simulink model "A_Justo_SCHFV_slx_Track"  (R2019a)
settings: Solver=VariableStepAuto  StartTime=0.0  StopTime=tfinal  MaxStep=maxstepsize  RelTol=1e-3  EnableMultiTasking=on
values from neighbouring files (symbols this model uses):
  acc1 = 0    [A_Justo_SCHFV_m_IV.m]    (also in A_Justo_SCHFV_m_Track.m)
  acc2 = 0    [A_Justo_SCHFV_m_IV.m]    (also in A_Justo_SCHFV_m_Track.m)
  add_u_1 = zeros(N,1); add_u_1(acc1) = 1    [A_Justo_SCHFV_m_Track.m]
  add_u_2 = zeros(N,1)    [A_Justo_SCHFV_m_Track.m]
  aini = 0    [A_Justo_SCHFV_m_UFHDV_Design.m]
  B = [0; 0; 0; 0; 1/Tau_A]    [A_Justo_SCHFV_m_Control_Sensitivity.m]    (also in A_Justo_SCHFV_m_UFHDV_Design.m; TransferFunctionPROP.m)
  IDM_Amax = IDM_Amax(acc1+n1,acc1+n1)    [TransferFunctionPROP.m]
  IDM_Bmax = IDM_Bmax(acc1+n1,acc1+n1)    [TransferFunctionPROP.m]
  IDM_Delta = IDM_Delta(acc1+n1)    [TransferFunctionPROP.m]
  IDM_H0 = IDM_H0(acc1+n1)    [TransferFunctionPROP.m]
  IDM_T = normrnd(IDM_t,IDM_ts)    [A_Justo_SCHFV_m_Control_Sensitivity.m]    (also in A_Justo_SCHFV_m_Track.m = IDM_Tind; A_Justo_SCHFV_m_UFHDV_Design.m; TransferFunctionPROP.m = IDM_T(acc1+n1,acc1+n1))
  IDM_V0 = IDM_V0(acc1+n1)    [TransferFunctionPROP.m]
  kgain = 0.02    [A_Justo_SCHFV_m_Track.m]    (also in A_Justo_SCHFV_m_UFHDV_Design.m)
  Lini = Lind    [A_Justo_SCHFV_m_Track.m]    (also in A_Justo_SCHFV_m_UFHDV_Design.m = sum(normrnd(l,ls,1,n)))
  N = 11    [A_Justo_SCHFV_m_IV.m]    (also in A_Justo_SCHFV_m_Track.m)
  n1 = 0    [A_Justo_SCHFV_m_IV.m]    (also in A_Justo_SCHFV_m_Track.m = 10)
  R = d/(2*pi)    (= 31.8309886184)    [A_Justo_SCHFV_m_IV.m]    (also in A_Justo_SCHFV_m_Track.m)
  Sacc = diag(isACC)    [A_Justo_SCHFV_m_Track.m]
  sep_a_A_1 = zeros(1,N); sep_a_A_1(acc1) = 1    [A_Justo_SCHFV_m_Track.m]
  sep_a_A_2 = zeros(1,N)    [A_Justo_SCHFV_m_Track.m]
  sep_a_H_1 = zeros(1,N); sep_a_H_1(acc1+n1) = 1    [A_Justo_SCHFV_m_Track.m]
  sep_a_H_2 = zeros(1,N)    [A_Justo_SCHFV_m_Track.m]
  sep_h_H_1 = zeros(1,N); sep_h_H_1(acc1+1) = 1    [A_Justo_SCHFV_m_Track.m]
  sep_h_H_2 = zeros(1,N)    [A_Justo_SCHFV_m_Track.m]
  sep_v_A_1 = zeros(1,N); sep_v_A_1(acc1) = 1    [A_Justo_SCHFV_m_Track.m]
  sep_v_A_2 = zeros(1,N)    [A_Justo_SCHFV_m_Track.m]
  sep_v_H_1 = zeros(1,N); sep_v_H_1(acc1+n1) = 1    [A_Justo_SCHFV_m_Track.m]
  sep_v_H_2 = zeros(1,N)    [A_Justo_SCHFV_m_Track.m]
  Sidm = diag(isIDM)    [A_Justo_SCHFV_m_IV.m]    (also in A_Justo_SCHFV_m_Track.m)
  Smit = diag(isMIT)    [A_Justo_SCHFV_m_IV.m]    (also in A_Justo_SCHFV_m_Track.m)
  T_s_0 = 60    [A_Justo_SCHFV_m_Track.m]
  v_r_0 = 30/3.6    (= 8.33333333333)    [A_Justo_SCHFV_m_Control_Sensitivity.m]    (also in A_Justo_SCHFV_m_Track.m = 5.55555555556; A_Justo_SCHFV_m_UFHDV_Design.m = 2.77777777778)
  vini = 0    [A_Justo_SCHFV_m_UFHDV_Design.m]
undefined symbols (not defined in the file or in its folder): Bv, IDM_iSqab, iTau, MITSIM_a_Free_bra_high, MITSIM_a_Free_bra_low, MITSIM_a_Free_bra_mid, MITSIM_a_Free_bra_midhigh, MITSIM_a_Free_bra_midlow, MITSIM_a_Free_thr_high, MITSIM_a_Free_thr_low, MITSIM_a_Free_thr_mid, MITSIM_Alpha_bra, MITSIM_Alpha_thr, MITSIM_Beta_bra, MITSIM_Beta_thr, MITSIM_Gamma_bra, MITSIM_Gamma_thr, MITSIM_T_lower, MITSIM_T_upper, Tau, thini
settings Model: Creator=arnaudoria  LastModifiedBy=Sander
settings DataIOCC: LimitDataPoints=on  ReturnWorkspaceOutputs=off
settings OptimizationCC: LifeSpan=inf
settings DebuggingCC: AllowSymbolicDim=off  SFUnexpectedBacktrackingDiag=warning  SFNoUnconditionalDefaultTransitionDiag=warning  SFExecutionAtInitializationDiag=none  ArithmeticOperatorsInVariantConditions=warning
settings ModelReferenceCC: PropagateSignalLabelsOutOfModel=off
settings SFSimCC: SimUseLocalCustomCode=off
settings RTWCC: RTWUseLocalCustomCode=off
settings CodeAppCC: StateflowObjectComments=on
settings GRTTargetCC: TargetLangStandard=C89/C90 (ANSI)
settings ConfigComp: CovMetricSettings=dw  CovHtmlReporting=on  CovSaveCumulativeToWorkspaceVar=on  CovSaveSingleToWorkspaceVar=on  CovExternalEMLEnable=off

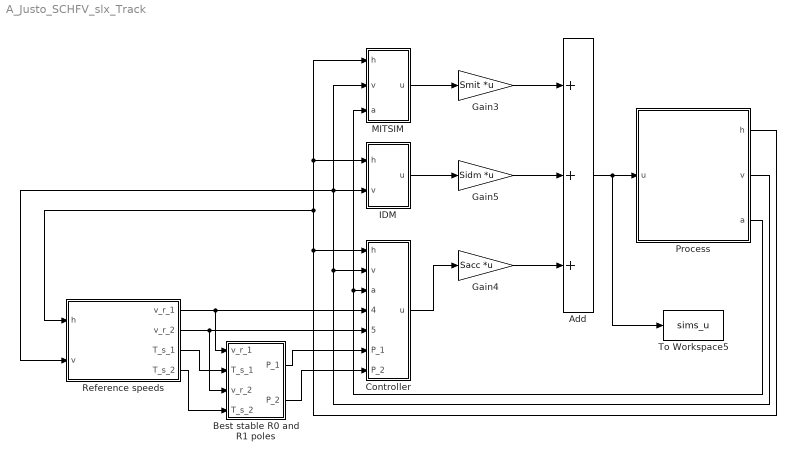
== system A_Justo_SCHFV_slx_Track ==
  Add : Sum  Inputs=+++
  Best stable R0 and R1 poles : Subsystem
  Controller : Subsystem
  Gain3 : Gain  Gain=Smit  Multiplication=Matrix(K*u)
  Gain4 : Gain  Gain=Sacc  Multiplication=Matrix(K*u)
  Gain5 : Gain  Gain=Sidm  Multiplication=Matrix(K*u)
  IDM : Subsystem
  MITSIM : Subsystem
  Process : Subsystem
  Reference speeds : Subsystem
  To Workspace5 : ToWorkspace  VariableName=sims_u  SampleTime=-1
  wires:
  Process/1(h) -> Reference speeds/1(h), IDM/1(h), MITSIM/1(h), Controller/1(h)
  Process/2(v) -> Reference speeds/2(v), MITSIM/2(v), IDM/2(v), Controller/2(v)
  Process/3(a) -> MITSIM/3(a), Controller/3(a)
  Controller/1(u) -> Gain4/1
  Gain4/1 -> Add/3
  Add/1 -> Process/1(u), To Workspace5/1
  Gain5/1 -> Add/2
  IDM/1(u) -> Gain5/1
  MITSIM/1(u) -> Gain3/1
  Gain3/1 -> Add/1
  Reference speeds/1(v_r_1) -> Controller/4(v_r_1), Best stable R0 and R1 poles/1(v_r_1)
  Best stable R0 and R1 poles/1(P_1) -> Controller/6(P_1)
  Reference speeds/2(v_r_2) -> Best stable R0 and R1 poles/3(v_r_2), Controller/5(v_r_2)
  Best stable R0 and R1 poles/2(P_2) -> Controller/7(P_2)
  Reference speeds/3(T_s_1) -> Best stable R0 and R1 poles/2(T_s_1)
  Reference speeds/4(T_s_2) -> Best stable R0 and R1 poles/4(T_s_2)

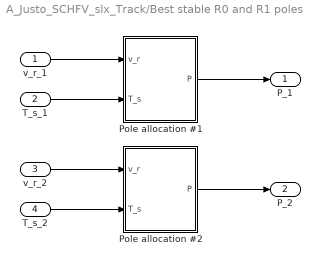
== system A_Justo_SCHFV_slx_Track/Best stable R0 and R1 poles ==
  v_r_1 : Inport
  T_s_1 : Inport  Port=2
  v_r_2 : Inport  Port=3
  T_s_2 : Inport  Port=4
  Pole allocation #1 : MATLAB Function  TreatAsAtomicUnit=on
  Pole allocation #2 : MATLAB Function  TreatAsAtomicUnit=on
  P_1 : Outport
  P_2 : Outport  Port=2
  wires:
  v_r_1/1 -> Pole allocation #1/1(v_r)
  Pole allocation #1/1(P) -> P_1/1
  T_s_1/1 -> Pole allocation #1/2(T_s)
  Pole allocation #2/1(P) -> P_2/1
  T_s_2/1 -> Pole allocation #2/2(T_s)
  v_r_2/1 -> Pole allocation #2/1(v_r)

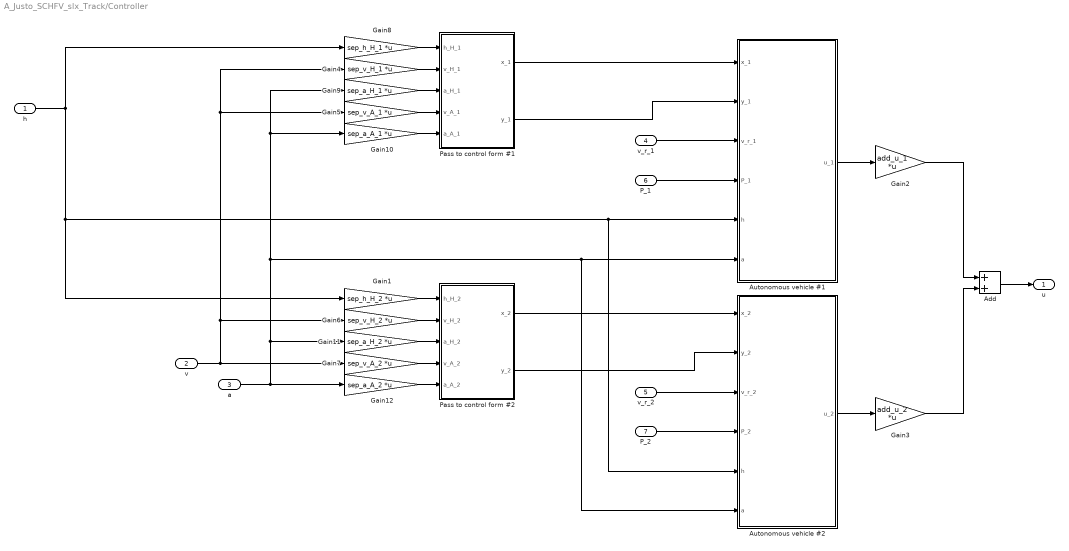
== system A_Justo_SCHFV_slx_Track/Controller ==
  h : Inport
  v : Inport  Port=2
  a : Inport  Port=3
  v_r_1 : Inport  Port=4
  v_r_2 : Inport  Port=5
  P_1 : Inport  Port=6
  P_2 : Inport  Port=7
  Add : Sum
  Autonomous vehicle #1 : Subsystem
  Autonomous vehicle #2 : Subsystem
  Gain1 : Gain  Gain=sep_h_H_2  Multiplication=Matrix(K*u)
  Gain10 : Gain  Gain=sep_a_A_1  Multiplication=Matrix(K*u)
  Gain11 : Gain  Gain=sep_a_H_2  Multiplication=Matrix(K*u)
  Gain12 : Gain  Gain=sep_a_A_2  Multiplication=Matrix(K*u)
  Gain2 : Gain  Gain=add_u_1  Multiplication=Matrix(K*u)
  Gain3 : Gain  Gain=add_u_2  Multiplication=Matrix(K*u)
  Gain4 : Gain  Gain=sep_v_H_1  Multiplication=Matrix(K*u)
  Gain5 : Gain  Gain=sep_v_A_1  Multiplication=Matrix(K*u)
  Gain6 : Gain  Gain=sep_v_H_2  Multiplication=Matrix(K*u)
  Gain7 : Gain  Gain=sep_v_A_2  Multiplication=Matrix(K*u)
  Gain8 : Gain  Gain=sep_h_H_1  Multiplication=Matrix(K*u)
  Gain9 : Gain  Gain=sep_a_H_1  Multiplication=Matrix(K*u)
  Pass to control form #1 : Subsystem
  Pass to control form #2 : Subsystem
  u : Outport
  wires:
  Gain2/1 -> Add/1
  Gain3/1 -> Add/2
  Add/1 -> u/1
  h/1 -> Gain1/1, Autonomous vehicle #2/5(h), Autonomous vehicle #1/5(h), Gain8/1
  v/1 -> Gain5/1, Gain4/1, Gain6/1, Gain7/1
  a/1 -> Autonomous vehicle #2/6(a), Autonomous vehicle #1/6(a), Gain9/1, Gain10/1, Gain11/1, Gain12/1
  Autonomous vehicle #1/1(u_1) -> Gain2/1
  Gain8/1 -> Pass to control form #1/1(h_H_1)
  Gain1/1 -> Pass to control form #2/1(h_H_2)
  Gain4/1 -> Pass to control form #1/2(v_H_1)
  Gain5/1 -> Pass to control form #1/4(v_A_1)
  Gain6/1 -> Pass to control form #2/2(v_H_2)
  Gain7/1 -> Pass to control form #2/4(v_A_2)
  Gain9/1 -> Pass to control form #1/3(a_H_1)
  Gain10/1 -> Pass to control form #1/5(a_A_1)
  Gain11/1 -> Pass to control form #2/3(a_H_2)
  Gain12/1 -> Pass to control form #2/5(a_A_2)
  Pass to control form #1/1(x_1) -> Autonomous vehicle #1/1(x_1)
  Pass to control form #1/2(y_1) -> Autonomous vehicle #1/2(y_1)
  Pass to control form #2/1(x_2) -> Autonomous vehicle #2/1(x_2)
  Pass to control form #2/2(y_2) -> Autonomous vehicle #2/2(y_2)
  P_1/1 -> Autonomous vehicle #1/4(P_1)
  v_r_2/1 -> Autonomous vehicle #2/3(v_r_2)
  P_2/1 -> Autonomous vehicle #2/4(P_2)
  v_r_1/1 -> Autonomous vehicle #1/3(v_r_1)
  Autonomous vehicle #2/1(u_2) -> Gain3/1

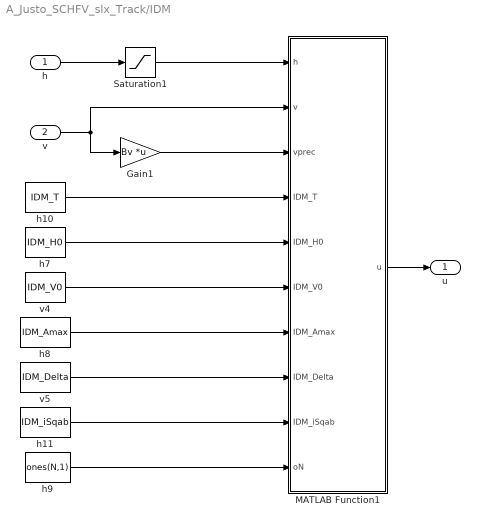
== system A_Justo_SCHFV_slx_Track/IDM ==
  h : Inport
  v : Inport  Port=2
  Gain1 : Gain  Gain=Bv  Multiplication=Matrix(K*u)
  MATLAB Function1 : MATLAB Function  TreatAsAtomicUnit=on
  Saturation1 : Saturate  UpperLimit=inf  LowerLimit=0.1
  h10 : Constant  Value=IDM_T
  h11 : Constant  Value=IDM_iSqab
  h7 : Constant  Value=IDM_H0
  h8 : Constant  Value=IDM_Amax
  h9 : Constant  Value=ones(N,1)
  v4 : Constant  Value=IDM_V0
  v5 : Constant  Value=IDM_Delta
  u : Outport
  wires:
  v4/1 -> MATLAB Function1/6(IDM_V0)
  h7/1 -> MATLAB Function1/5(IDM_H0)
  h/1 -> Saturation1/1
  v5/1 -> MATLAB Function1/8(IDM_Delta)
  Saturation1/1 -> MATLAB Function1/1(h)
  h9/1 -> MATLAB Function1/10(oN)
  Gain1/1 -> MATLAB Function1/3(vprec)
  h10/1 -> MATLAB Function1/4(IDM_T)
  MATLAB Function1/1(u) -> u/1
  v/1 -> Gain1/1, MATLAB Function1/2(v)
  h11/1 -> MATLAB Function1/9(IDM_iSqab)
  h8/1 -> MATLAB Function1/7(IDM_Amax)

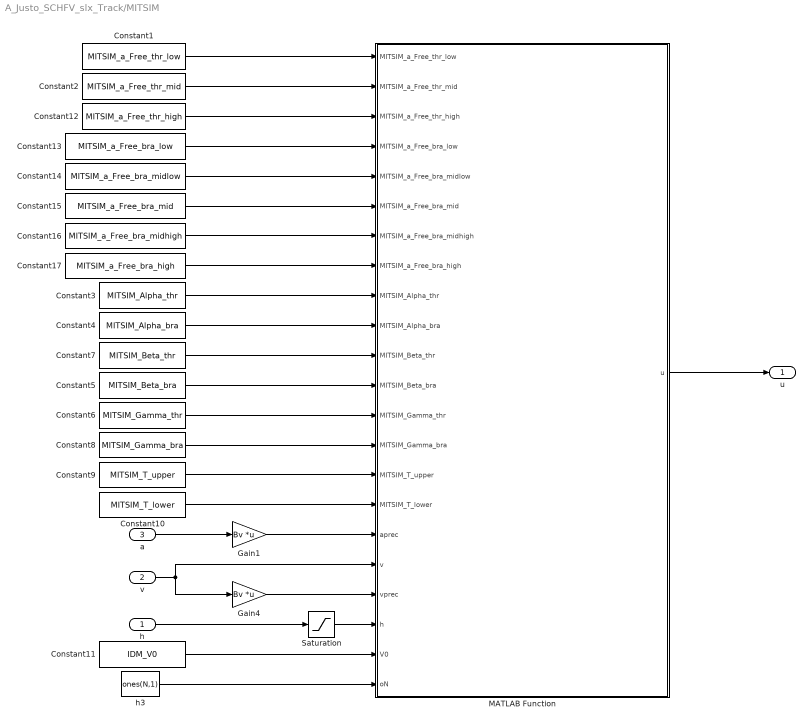
== system A_Justo_SCHFV_slx_Track/MITSIM ==
  h : Inport
  v : Inport  Port=2
  a : Inport  Port=3
  Constant1 : Constant  Value=MITSIM_a_Free_thr_low
  Constant10 : Constant  Value=MITSIM_T_lower
  Constant11 : Constant  Value=IDM_V0
  Constant12 : Constant  Value=MITSIM_a_Free_thr_high
  Constant13 : Constant  Value=MITSIM_a_Free_bra_low
  Constant14 : Constant  Value=MITSIM_a_Free_bra_midlow
  Constant15 : Constant  Value=MITSIM_a_Free_bra_mid
  Constant16 : Constant  Value=MITSIM_a_Free_bra_midhigh
  Constant17 : Constant  Value=MITSIM_a_Free_bra_high
  Constant2 : Constant  Value=MITSIM_a_Free_thr_mid
  Constant3 : Constant  Value=MITSIM_Alpha_thr
  Constant4 : Constant  Value=MITSIM_Alpha_bra
  Constant5 : Constant  Value=MITSIM_Beta_bra
  Constant6 : Constant  Value=MITSIM_Gamma_thr
  Constant7 : Constant  Value=MITSIM_Beta_thr
  Constant8 : Constant  Value=MITSIM_Gamma_bra
  Constant9 : Constant  Value=MITSIM_T_upper
  Gain1 : Gain  Gain=Bv  Multiplication=Matrix(K*u)
  Gain4 : Gain  Gain=Bv  Multiplication=Matrix(K*u)
  MATLAB Function : MATLAB Function  TreatAsAtomicUnit=on
  Saturation : Saturate  UpperLimit=inf  LowerLimit=0.1
  h3 : Constant  Value=ones(N,1)
  u : Outport
  wires:
  Saturation/1 -> MATLAB Function/20(h)
  h/1 -> Saturation/1
  MATLAB Function/1(u) -> u/1
  Gain4/1 -> MATLAB Function/19(vprec)
  v/1 -> Gain4/1, MATLAB Function/18(v)
  Constant1/1 -> MATLAB Function/1(MITSIM_a_Free_thr_low)
  Constant2/1 -> MATLAB Function/2(MITSIM_a_Free_thr_mid)
  Constant3/1 -> MATLAB Function/9(MITSIM_Alpha_thr)
  h3/1 -> MATLAB Function/22(oN)
  a/1 -> Gain1/1
  Gain1/1 -> MATLAB Function/17(aprec)
  Constant4/1 -> MATLAB Function/10(MITSIM_Alpha_bra)
  Constant7/1 -> MATLAB Function/11(MITSIM_Beta_thr)
  Constant5/1 -> MATLAB Function/12(MITSIM_Beta_bra)
  Constant6/1 -> MATLAB Function/13(MITSIM_Gamma_thr)
  Constant8/1 -> MATLAB Function/14(MITSIM_Gamma_bra)
  Constant9/1 -> MATLAB Function/15(MITSIM_T_upper)
  Constant10/1 -> MATLAB Function/16(MITSIM_T_lower)
  Constant11/1 -> MATLAB Function/21(V0)
  Constant12/1 -> MATLAB Function/3(MITSIM_a_Free_thr_high)
  Constant13/1 -> MATLAB Function/4(MITSIM_a_Free_bra_low)
  Constant14/1 -> MATLAB Function/5(MITSIM_a_Free_bra_midlow)
  Constant15/1 -> MATLAB Function/6(MITSIM_a_Free_bra_mid)
  Constant16/1 -> MATLAB Function/7(MITSIM_a_Free_bra_midhigh)
  Constant17/1 -> MATLAB Function/8(MITSIM_a_Free_bra_high)

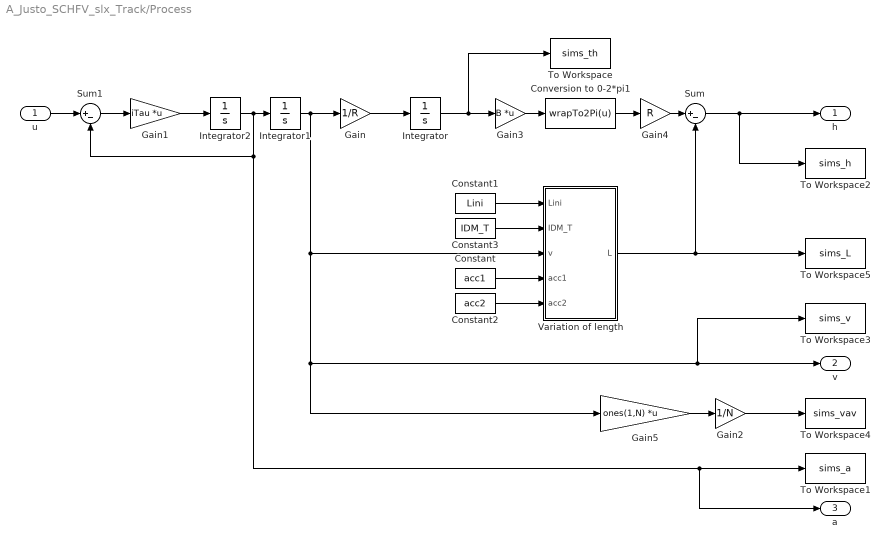
== system A_Justo_SCHFV_slx_Track/Process ==
  u : Inport
  Constant : Constant  Value=acc1
  Constant1 : Constant  Value=Lini
  Constant2 : Constant  Value=acc2
  Constant3 : Constant  Value=IDM_T
  Conversion to 0-2*pi1 : MATLABFcn  MATLABFcn=wrapTo2Pi(u)
  Gain : Gain  Gain=1/R
  Gain1 : Gain  Gain=iTau  Multiplication=Matrix(K*u)
  Gain2 : Gain  Gain=1/N
  Gain3 : Gain  Gain=B  Multiplication=Matrix(K*u)
  Gain4 : Gain  Gain=R
  Gain5 : Gain  Gain=ones(1,N)  Multiplication=Matrix(K*u)
  Integrator : Integrator  InitialCondition=thini  WrapState=on  WrappedStateUpperValue=2*pi  WrappedStateLowerValue=0
  Integrator1 : Integrator  InitialCondition=vini  LimitOutput=on  UpperSaturationLimit=+inf  LowerSaturationLimit=0  WrappedStateUpperValue=2*pi  WrappedStateLowerValue=0
  Integrator2 : Integrator  InitialCondition=aini  UpperSaturationLimit=1  WrappedStateUpperValue=2*pi  WrappedStateLowerValue=0
  Sum : Sum  Inputs=|+-
  Sum1 : Sum  Inputs=|+-
  To Workspace : ToWorkspace  VariableName=sims_th  SampleTime=-1
  To Workspace1 : ToWorkspace  VariableName=sims_a  SampleTime=-1
  To Workspace2 : ToWorkspace  VariableName=sims_h  SampleTime=-1
  To Workspace3 : ToWorkspace  VariableName=sims_v  SampleTime=-1
  To Workspace4 : ToWorkspace  VariableName=sims_vav  SampleTime=-1
  To Workspace5 : ToWorkspace  VariableName=sims_L  SampleTime=-1
  Variation of length : MATLAB Function  TreatAsAtomicUnit=on
  h : Outport
  v : Outport  Port=2
  a : Outport  Port=3
  wires:
  Gain/1 -> Integrator/1
  Gain3/1 -> Conversion to 0-2*pi1/1
  Gain4/1 -> Sum/1
  Sum/1 -> To Workspace2/1, h/1
  u/1 -> Sum1/1
  Integrator1/1 -> Gain5/1, To Workspace3/1, v/1, Variation of length/3(v), Gain/1
  Integrator2/1 -> To Workspace1/1, a/1, Sum1/2, Integrator1/1
  Gain1/1 -> Integrator2/1
  Sum1/1 -> Gain1/1
  Integrator/1 -> To Workspace/1, Gain3/1
  Conversion to 0-2*pi1/1 -> Gain4/1
  Gain5/1 -> Gain2/1
  Gain2/1 -> To Workspace4/1
  Constant/1 -> Variation of length/4(acc1)
  Constant2/1 -> Variation of length/5(acc2)
  Variation of length/1(L) -> Sum/2, To Workspace5/1
  Constant3/1 -> Variation of length/2(IDM_T)
  Constant1/1 -> Variation of length/1(Lini)

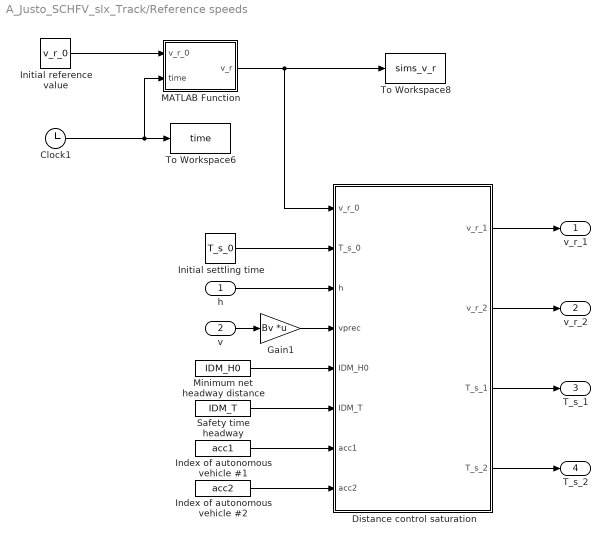
== system A_Justo_SCHFV_slx_Track/Reference speeds ==
  h : Inport
  v : Inport  Port=2
  Clock1 : Clock
  Distance control saturation : MATLAB Function  TreatAsAtomicUnit=on
  Gain1 : Gain  Gain=Bv  Multiplication=Matrix(K*u)
  Index of autonomous vehicle #1 : Constant  Value=acc1
  Index of autonomous vehicle #2 : Constant  Value=acc2
  Initial reference value : Constant  Value=v_r_0
  Initial settling time : Constant  Value=T_s_0
  MATLAB Function : MATLAB Function  TreatAsAtomicUnit=on
  Minimum net headway distance : Constant  Value=IDM_H0
  Safety time headway : Constant  Value=IDM_T
  To Workspace6 : ToWorkspace  VariableName=time  SampleTime=-1
  To Workspace8 : ToWorkspace  VariableName=sims_v_r  SampleTime=-1
  v_r_1 : Outport
  v_r_2 : Outport  Port=2
  T_s_1 : Outport  Port=3
  T_s_2 : Outport  Port=4
  wires:
  Clock1/1 -> To Workspace6/1, MATLAB Function/2(time)
  Initial reference value/1 -> MATLAB Function/1(v_r_0)
  h/1 -> Distance control saturation/3(h)
  Minimum net headway distance/1 -> Distance control saturation/5(IDM_H0)
  Safety time headway/1 -> Distance control saturation/6(IDM_T)
  Gain1/1 -> Distance control saturation/4(vprec)
  v/1 -> Gain1/1
  MATLAB Function/1(v_r) -> Distance control saturation/1(v_r_0), To Workspace8/1
  Index of autonomous vehicle #1/1 -> Distance control saturation/7(acc1)
  Index of autonomous vehicle #2/1 -> Distance control saturation/8(acc2)
  Distance control saturation/4(T_s_2) -> T_s_2/1
  Distance control saturation/3(T_s_1) -> T_s_1/1
  Distance control saturation/1(v_r_1) -> v_r_1/1
  Distance control saturation/2(v_r_2) -> v_r_2/1
  Initial settling time/1 -> Distance control saturation/2(T_s_0)

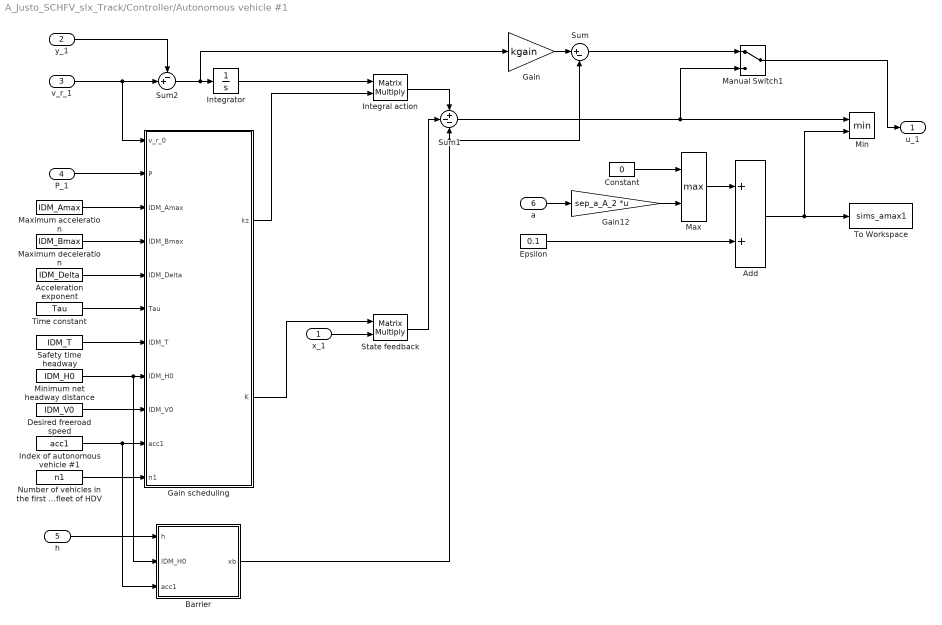
== system A_Justo_SCHFV_slx_Track/Controller/Autonomous vehicle #1 ==
  x_1 : Inport
  y_1 : Inport  Port=2
  v_r_1 : Inport  Port=3
  P_1 : Inport  Port=4
  h : Inport  Port=5
  a : Inport  Port=6
  Acceleration exponent : Constant  Value=IDM_Delta
  Add : Sum
  Barrier : MATLAB Function  TreatAsAtomicUnit=on
  Constant : Constant  Value=0
  Desired freeroad speed : Constant  Value=IDM_V0
  Epsilon : Constant  Value=0.1
  Gain : Gain  Gain=kgain
  Gain scheduling : MATLAB Function  TreatAsAtomicUnit=on
  Gain12 : Gain  Gain=sep_a_A_2  Multiplication=Matrix(K*u)
  Index of autonomous vehicle #1 : Constant  Value=acc1
  Integral action : Product  Multiplication=Matrix(*)
  Integrator : Integrator
  Manual Switch1 : ManualSwitch
  Max : MinMax  Function=max  Inputs=2
  Maximum acceleration : Constant  Value=IDM_Amax
  Maximum deceleration : Constant  Value=IDM_Bmax
  Min : MinMax  Inputs=2
  Minimum net headway distance : Constant  Value=IDM_H0
  Number of vehicles in the first fleet of HDV : Constant  Value=n1
  Safety time headway : Constant  Value=IDM_T
  State feedback : Product  Multiplication=Matrix(*)
  Sum : Sum  Inputs=|+-
  Sum1 : Sum  Inputs=+--
  Sum2 : Sum  Inputs=-+|
  Time constant : Constant  Value=Tau
  To Workspace : ToWorkspace  VariableName=sims_amax1  SampleTime=-1
  u_1 : Outport
  wires:
  v_r_1/1 -> Sum2/2, Gain scheduling/1(v_r_0)
  Acceleration exponent/1 -> Gain scheduling/5(IDM_Delta)
  Time constant/1 -> Gain scheduling/6(Tau)
  Maximum acceleration/1 -> Gain scheduling/3(IDM_Amax)
  Maximum deceleration/1 -> Gain scheduling/4(IDM_Bmax)
  Minimum net headway distance/1 -> Barrier/2(IDM_H0), Gain scheduling/8(IDM_H0)
  Integral action/1 -> Sum1/1
  Sum2/1 -> Gain/1, Integrator/1
  Safety time headway/1 -> Gain scheduling/7(IDM_T)
  Gain scheduling/1(kz) -> Integral action/2
  Gain scheduling/2(K) -> State feedback/1
  Desired freeroad speed/1 -> Gain scheduling/9(IDM_V0)
  State feedback/1 -> Sum1/2
  P_1/1 -> Gain scheduling/2(P)
  y_1/1 -> Sum2/1
  x_1/1 -> State feedback/2
  Index of autonomous vehicle #1/1 -> Gain scheduling/10(acc1), Barrier/3(acc1)
  Number of vehicles in the first fleet of HDV/1 -> Gain scheduling/11(n1)
  h/1 -> Barrier/1(h)
  Barrier/1(xb) -> Sum/2, Sum1/3
  a/1 -> Gain12/1
  Sum1/1 -> Manual Switch1/2, Min/1
  Gain12/1 -> Max/2
  Constant/1 -> Max/1
  Max/1 -> Add/1
  Epsilon/1 -> Add/2
  Add/1 -> Min/2, To Workspace/1
  Integrator/1 -> Integral action/1
  Manual Switch1/1 -> u_1/1
  Sum/1 -> Manual Switch1/1
  Gain/1 -> Sum/1

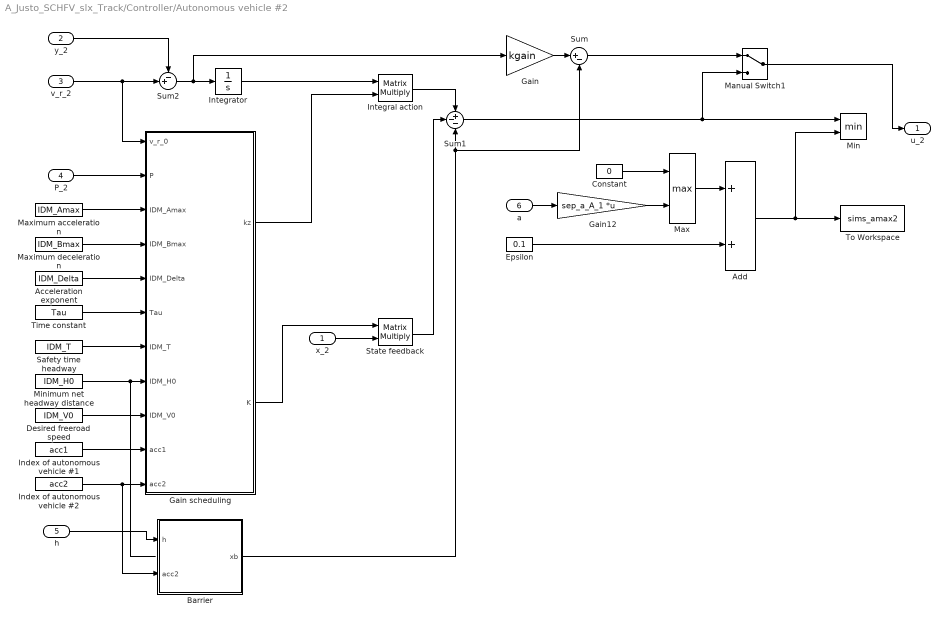
== system A_Justo_SCHFV_slx_Track/Controller/Autonomous vehicle #2 ==
  x_2 : Inport
  y_2 : Inport  Port=2
  v_r_2 : Inport  Port=3
  P_2 : Inport  Port=4
  h : Inport  Port=5
  a : Inport  Port=6
  Acceleration exponent : Constant  Value=IDM_Delta
  Add : Sum
  Barrier : MATLAB Function  TreatAsAtomicUnit=on
  Constant : Constant  Value=0
  Desired freeroad speed : Constant  Value=IDM_V0
  Epsilon : Constant  Value=0.1
  Gain : Gain  Gain=kgain
  Gain scheduling : MATLAB Function  TreatAsAtomicUnit=on
  Gain12 : Gain  Gain=sep_a_A_1  Multiplication=Matrix(K*u)
  Index of autonomous vehicle #1 : Constant  Value=acc1
  Index of autonomous vehicle #2 : Constant  Value=acc2
  Integral action : Product  Multiplication=Matrix(*)
  Integrator : Integrator
  Manual Switch1 : ManualSwitch
  Max : MinMax  Function=max  Inputs=2
  Maximum acceleration : Constant  Value=IDM_Amax
  Maximum deceleration : Constant  Value=IDM_Bmax
  Min : MinMax  Inputs=2
  Minimum net headway distance : Constant  Value=IDM_H0
  Safety time headway : Constant  Value=IDM_T
  State feedback : Product  Multiplication=Matrix(*)
  Sum : Sum  Inputs=|+-
  Sum1 : Sum  Inputs=+--
  Sum2 : Sum  Inputs=-+|
  Time constant : Constant  Value=Tau
  To Workspace : ToWorkspace  VariableName=sims_amax2  SampleTime=-1
  u_2 : Outport
  wires:
  x_2/1 -> State feedback/2
  Integrator/1 -> Integral action/1
  State feedback/1 -> Sum1/2
  Gain scheduling/2(K) -> State feedback/1
  Gain scheduling/1(kz) -> Integral action/2
  v_r_2/1 -> Gain scheduling/1(v_r_0), Sum2/2
  y_2/1 -> Sum2/1
  Integral action/1 -> Sum1/1
  Desired freeroad speed/1 -> Gain scheduling/9(IDM_V0)
  Minimum net headway distance/1 -> Gain scheduling/8(IDM_H0)
  Safety time headway/1 -> Gain scheduling/7(IDM_T)
  Maximum deceleration/1 -> Gain scheduling/4(IDM_Bmax)
  Time constant/1 -> Gain scheduling/6(Tau)
  Acceleration exponent/1 -> Gain scheduling/5(IDM_Delta)
  Index of autonomous vehicle #1/1 -> Gain scheduling/10(acc1)
  P_2/1 -> Gain scheduling/2(P)
  Maximum acceleration/1 -> Gain scheduling/3(IDM_Amax)
  Index of autonomous vehicle #2/1 -> Barrier/2(acc2), Gain scheduling/11(acc2)
  h/1 -> Barrier/1(h)
  a/1 -> Gain12/1
  Max/1 -> Add/1
  Constant/1 -> Max/1
  Epsilon/1 -> Add/2
  Gain12/1 -> Max/2
  Add/1 -> To Workspace/1, Min/2
  Manual Switch1/1 -> u_2/1
  Sum2/1 -> Gain/1, Integrator/1
  Sum1/1 -> Manual Switch1/2, Min/1
  Gain/1 -> Sum/1
  Barrier/1(xb) -> Sum/2, Sum1/3
  Sum/1 -> Manual Switch1/1

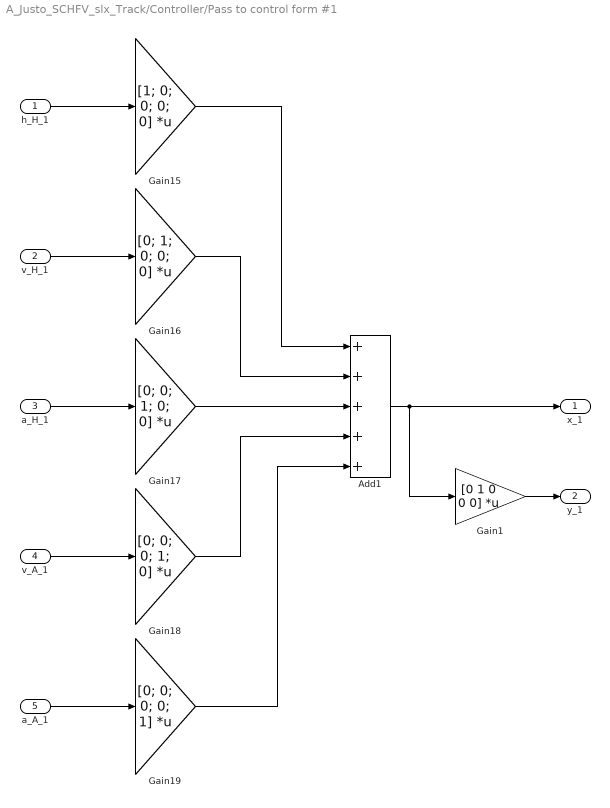
== system A_Justo_SCHFV_slx_Track/Controller/Pass to control form #1 ==
  h_H_1 : Inport
  v_H_1 : Inport  Port=2
  a_H_1 : Inport  Port=3
  v_A_1 : Inport  Port=4
  a_A_1 : Inport  Port=5
  Add1 : Sum  Inputs=+++++
  Gain1 : Gain  Gain=[0 1 0 0 0]  Multiplication=Matrix(K*u)
  Gain15 : Gain  Gain=[1; 0; 0; 0; 0]  Multiplication=Matrix(K*u)
  Gain16 : Gain  Gain=[0; 1; 0; 0; 0]  Multiplication=Matrix(K*u)
  Gain17 : Gain  Gain=[0; 0; 1; 0; 0]  Multiplication=Matrix(K*u)
  Gain18 : Gain  Gain=[0; 0; 0; 1; 0]  Multiplication=Matrix(K*u)
  Gain19 : Gain  Gain=[0; 0; 0; 0; 1]  Multiplication=Matrix(K*u)
  x_1 : Outport
  y_1 : Outport  Port=2
  wires:
  Gain15/1 -> Add1/1
  Gain16/1 -> Add1/2
  Gain18/1 -> Add1/4
  Gain19/1 -> Add1/5
  Gain17/1 -> Add1/3
  Add1/1 -> Gain1/1, x_1/1
  v_H_1/1 -> Gain16/1
  h_H_1/1 -> Gain15/1
  a_H_1/1 -> Gain17/1
  v_A_1/1 -> Gain18/1
  a_A_1/1 -> Gain19/1
  Gain1/1 -> y_1/1

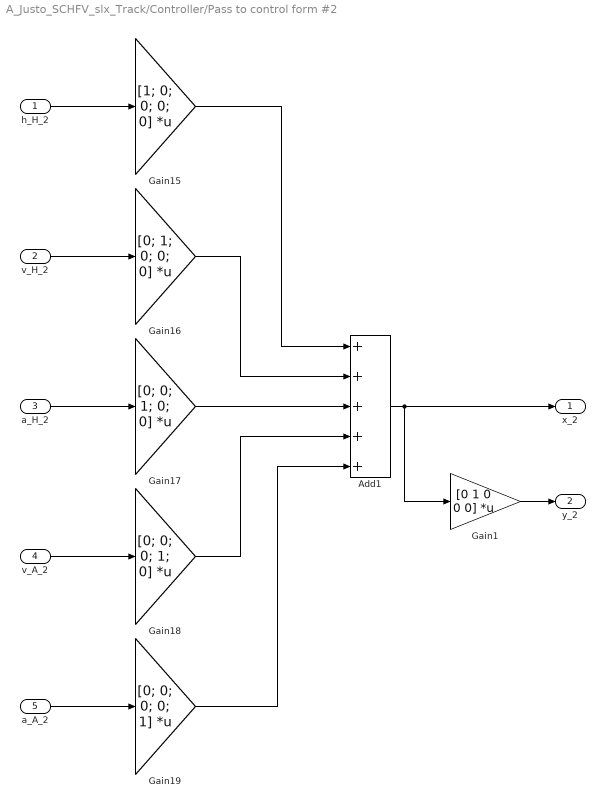
== system A_Justo_SCHFV_slx_Track/Controller/Pass to control form #2 ==
  h_H_2 : Inport
  v_H_2 : Inport  Port=2
  a_H_2 : Inport  Port=3
  v_A_2 : Inport  Port=4
  a_A_2 : Inport  Port=5
  Add1 : Sum  Inputs=+++++
  Gain1 : Gain  Gain=[0 1 0 0 0]  Multiplication=Matrix(K*u)
  Gain15 : Gain  Gain=[1; 0; 0; 0; 0]  Multiplication=Matrix(K*u)
  Gain16 : Gain  Gain=[0; 1; 0; 0; 0]  Multiplication=Matrix(K*u)
  Gain17 : Gain  Gain=[0; 0; 1; 0; 0]  Multiplication=Matrix(K*u)
  Gain18 : Gain  Gain=[0; 0; 0; 1; 0]  Multiplication=Matrix(K*u)
  Gain19 : Gain  Gain=[0; 0; 0; 0; 1]  Multiplication=Matrix(K*u)
  x_2 : Outport
  y_2 : Outport  Port=2
  wires:
  Gain15/1 -> Add1/1
  Gain16/1 -> Add1/2
  Gain18/1 -> Add1/4
  Gain19/1 -> Add1/5
  Gain17/1 -> Add1/3
  v_H_2/1 -> Gain16/1
  h_H_2/1 -> Gain15/1
  a_H_2/1 -> Gain17/1
  v_A_2/1 -> Gain18/1
  a_A_2/1 -> Gain19/1
  Gain1/1 -> y_2/1
  Add1/1 -> Gain1/1, x_2/1

== matlab function A_Justo_SCHFV_slx_Track/Reference speeds/MATLAB Function ==
  data: v_r_0 input; v_r output; time input
function v_r = fcn(v_r_0, time)
v_r = v_r_0;
% if time < 100
%     v_r = 1*v_r_0;
% elseif time >=100 && time <200
%     v_r = 2*v_r_0;
% elseif time >=200 && time <300
%     v_r = 3*v_r_0;
% elseif time >=300 && time <400
%     v_r = 4*v_r_0;
% elseif time >=400 && time <500
%     v_r = 3*v_r_0;
% elseif time >=500 && time <600
%     v_r = 2*v_r_0;
% elseif time >=600 && time <700
%     v_r = 1*v_r_0;
% end
end

== matlab function A_Justo_SCHFV_slx_Track/Controller/Autonomous vehicle #2/Gain scheduling ==
  data: kz output; v_r_0 input; K output; P input; IDM_Amax input; IDM_Bmax input; IDM_Delta input; Tau input; IDM_T input; IDM_H0 input; IDM_V0 input; acc1 input; acc2 input
function [kz,K] = fcn(v_r_0,P,IDM_Amax,IDM_Bmax,IDM_Delta,Tau,IDM_T,IDM_H0,IDM_V0,acc1,acc2)

IDM_Amax = IDM_Amax(end,end);
IDM_Bmax = IDM_Bmax(end,end);
IDM_Delta = IDM_Delta(end);
Tau_H = Tau(end,end);
%Tau_A = Tau(acc2,acc2);
Tau_A = Tau_H;
eta = IDM_T(end,end);
IDM_T = IDM_T(end,end);
IDM_H0 = IDM_H0(end);
IDM_V0 = IDM_V0(end);

A31 = 2*IDM_Amax/Tau_H/(IDM_H0+v_r_0*IDM_T)*(1-(v_r_0/IDM_V0)^IDM_Delta)^(3/2);
A32 = -IDM_Amax/Tau_H*(IDM_Delta*v_r_0^(IDM_Delta-1)/IDM_V0^IDM_Delta+(v_r_0+2*IDM_T*sqrt(IDM_Amax*IDM_Bmax))/((IDM_H0+v_r_0*IDM_T)*sqrt(IDM_Amax*IDM_Bmax))*(1-(v_r_0/IDM_V0)^IDM_Delta));
A34 = IDM_Amax/Tau_H*v_r_0/((IDM_H0+v_r_0*IDM_T)*sqrt(IDM_Amax*IDM_Bmax))*(1-(v_r_0/IDM_V0)^IDM_Delta);

% Linearized system
A = [ 0    -1     -eta      1       0    0 ;...
      0     0       1       0       0    0 ;...
     A31   A32  -1/Tau_H   A34      0    0 ;...
      0     0       0       0       1    0 ;...
      0     0       0       0   -1/Tau_A 0 ;...
      0     1       0       0       0    0 ];
B = [0; 0; 0; 0; 1/Tau_A; 0];

% Controllability matrix
W_C = [B A*B A^2*B A^3*B A^4*B A^5*B];

% Desired polynomial
P_d = (A-P(1)*eye(6))*(A-P(2)*eye(6))*(A-P(3)*eye(6))*(A-P(4)*eye(6))...
    *(A-P(5)*eye(6))*(A-P(6)*eye(6));

% Ackermann's formula
Kack = [0 0 0 0 0 1]*(W_C\P_d);
Kack = real(Kack);

% Gains
kz = Kack(6); K = [Kack(1) Kack(2) Kack(3) Kack(4) Kack(5)];

end

== matlab function A_Justo_SCHFV_slx_Track/Process/Variation of length ==
  data: Lini input; IDM_T input; v input; L output; acc1 input; acc2 input
function L = fcn(Lini, IDM_T, v, acc1, acc2)
% Plausibility model when the fleet of human driven vehicles is IDM
L = Lini;
% L(acc1)   = Lini(acc1);
% L(acc1+1) = Lini(acc1+1) + IDM_T(acc1+1,acc1+1)*v(acc1+1);
% L(acc2)   = Lini(acc2);
% L(acc2+1) = Lini(acc2+1) + IDM_T(acc2+1,acc2+1)*v(acc2+1);
end

== matlab function A_Justo_SCHFV_slx_Track/Best stable R0 and R1 poles/Pole allocation #1 ==
  data: v_r input; P output; T_s input
function P = fcn(v_r, T_s) % He mirado en el gráfico una T_s que funcione bien, pero habría que calcularlo a partir de v_r
% Design of the control
M_p = 1e-10; %overshoot
sigma = 4/T_s; %real part of dominant pair
omega = -pi*sigma/log(M_p); %imaginary part of dominant pair
pDom = -sigma + 1i*omega;
pNeg1 = -21*sigma; pNeg2 = -22*sigma; pNeg3 = -23*sigma; pNeg4 = -24*sigma;
P = [pDom; conj(pDom); pNeg1; pNeg2; pNeg3; pNeg4];
%P = [-sigma; pNeg1; pNeg2; pNeg3; pNeg4; -25*sigma];
end

== matlab function A_Justo_SCHFV_slx_Track/MITSIM/MATLAB Function ==
  data: MITSIM_a_Free_thr_low input; MITSIM_a_Free_thr_mid input; MITSIM_a_Free_thr_high input; MITSIM_a_Free_bra_low input; MITSIM_a_Free_bra_midlow input; MITSIM_a_Free_bra_mid input; MITSIM_a_Free_bra_midhigh input; MITSIM_a_Free_bra_high input; MITSIM_Alpha_thr input; MITSIM_Alpha_bra input; MITSIM_Beta_thr input; MITSIM_Beta_bra input; MITSIM_Gamma_thr input; MITSIM_Gamma_bra input; MITSIM_T_upper input; MITSIM_T_lower input; aprec input; v input; vprec input; h input; V0 input; u output; oN input
function u = fcn(MITSIM_a_Free_thr_low, MITSIM_a_Free_thr_mid, ...
    MITSIM_a_Free_thr_high, MITSIM_a_Free_bra_low, ...
    MITSIM_a_Free_bra_midlow, MITSIM_a_Free_bra_mid, ...
    MITSIM_a_Free_bra_midhigh, MITSIM_a_Free_bra_high, MITSIM_Alpha_thr...
    , MITSIM_Alpha_bra, MITSIM_Beta_thr, MITSIM_Beta_bra, ...
MITSIM_Gamma_thr, MITSIM_Gamma_bra, MITSIM_T_upper, MITSIM_T_lower, ...
aprec, v, vprec, h, V0, oN)

if isempty(find(h<=0, 1))==0  % Display a message to show when some h is not positive
    error('Vehicles have crashed. Simulation has been stopped.')
end

hd_tm = h./v;

% Obtain the indexes that correspond to each regime
ind_free_thr_low = hd_tm>MITSIM_T_upper & v<V0 & v>12.192;
ind_free_thr_mid = hd_tm>MITSIM_T_upper & v<V0 & v<=12.192 & v>=6.096;
ind_free_thr_high = hd_tm>MITSIM_T_upper & v<V0 & v<6.096;
ind_free_zro = hd_tm>MITSIM_T_upper & v==V0;
ind_free_bra_low = hd_tm>MITSIM_T_upper & v>V0 & v>24.4;
ind_free_bra_midlow = hd_tm>MITSIM_T_upper & v>V0 & v>=18.3 & v<=24.4;
ind_free_bra_mid = hd_tm>MITSIM_T_upper & v>V0 & v>=12.2 & v<18.3;
ind_free_bra_midhigh = hd_tm>MITSIM_T_upper & v>V0 & v>=6.1 & v<12.2;
ind_free_bra_high = hd_tm>MITSIM_T_upper & v>V0 & v<6.1;

ind_fllw_thr = hd_tm>=MITSIM_T_lower & hd_tm<=MITSIM_T_upper & v<=vprec;
ind_fllw_bra = hd_tm>=MITSIM_T_lower & hd_tm<=MITSIM_T_upper & v>vprec;

ind_emer_thr_low = hd_tm<MITSIM_T_lower & v<=vprec & v>24.4;
ind_emer_thr_midlow = hd_tm<MITSIM_T_lower & v<=vprec & v>=18.3 & v<=24.4;
ind_emer_thr_mid = hd_tm<MITSIM_T_lower & v<=vprec & v>=12.2 & v<18.3;
ind_emer_thr_midhigh = hd_tm<MITSIM_T_lower & v<=vprec & v>=6.1 & v<12.2;
ind_emer_thr_high = hd_tm<MITSIM_T_lower & v<=vprec & v<6.1;
ind_emer_bra_low = hd_tm<MITSIM_T_lower & v>vprec & v>24.4;
ind_emer_bra_midlow = hd_tm<MITSIM_T_lower & v>vprec & v>=18.3 & v<=24.4;
ind_emer_bra_mid = hd_tm<MITSIM_T_lower & v>vprec & v>=12.2 & v<18.3;
ind_emer_bra_midhigh = hd_tm<MITSIM_T_lower & v>vprec & v>=6.1 & v<12.2;
ind_emer_bra_high = hd_tm<MITSIM_T_lower & v>vprec & v<6.1;

% Control
u=oN*0;
% Condition for avoiding numerical errors
v = v.*(v>0);

% MITSIM - Free driving
u(ind_free_thr_low) = MITSIM_a_Free_thr_low(ind_free_thr_low,...
    ind_free_thr_low)*oN(ind_free_thr_low);
u(ind_free_thr_mid) = MITSIM_a_Free_thr_mid(ind_free_thr_mid,...
    ind_free_thr_mid)*oN(ind_free_thr_mid);
u(ind_free_thr_high) = MITSIM_a_Free_thr_high(ind_free_thr_high,...
    ind_free_thr_high)*oN(ind_free_thr_high);
u(ind_free_zro) = 0*oN(ind_free_zro);
u(ind_free_bra_low) = MITSIM_a_Free_bra_low(ind_free_bra_low,...
    ind_free_bra_low)*oN(ind_free_bra_low);
u(ind_free_bra_midlow) = MITSIM_a_Free_bra_midlow(ind_free_bra_midlow,...
    ind_free_bra_midlow)*oN(ind_free_bra_midlow);
u(ind_free_bra_mid) = MITSIM_a_Free_bra_mid(ind_free_bra_mid,...
    ind_free_bra_mid)*oN(ind_free_bra_mid);
u(ind_free_bra_midhigh) = MITSIM_a_Free_bra_midhigh(ind_free_bra_midhigh,...
    ind_free_bra_midhigh)*oN(ind_free_bra_midhigh);
u(ind_free_bra_high) = MITSIM_a_Free_bra_high(ind_free_bra_high,...
    ind_free_bra_high)*oN(ind_free_bra_high);

% MITSIM - Following regime
u(ind_fllw_thr) = MITSIM_Alpha_thr(ind_fllw_thr,ind_fllw_thr)*...
    (v(ind_fllw_thr).^MITSIM_Beta_thr(ind_fllw_thr).*...
    (vprec(ind_fllw_thr)-v(ind_fllw_thr))./h(ind_fllw_thr).^...
    MITSIM_Gamma_thr(ind_fllw_thr));
u(ind_fllw_bra) = MITSIM_Alpha_bra(ind_fllw_bra,ind_fllw_bra)*...
    (v(ind_fllw_bra).^MITSIM_Beta_bra(ind_fllw_bra).*...
    (vprec(ind_fllw_bra)-v(ind_fllw_bra))./h(ind_fllw_bra).^...
    MITSIM_Gamma_bra(ind_fllw_bra));

% MITSIM - Emergency brake
u(ind_emer_thr_low) = min(MITSIM_a_Free_bra_low(ind_emer_thr_low,...
    ind_emer_thr_low)*oN(ind_emer_thr_low),aprec(ind_emer_thr_low)...
    +0.25*MITSIM_a_Free_bra_low(ind_emer_thr_low,ind_emer_thr_low)...
    *oN(ind_emer_thr_low));
u(ind_emer_thr_midlow) = min(MITSIM_a_Free_bra_midlow(ind_emer_thr_midlow,...
    ind_emer_thr_midlow)*oN(ind_emer_thr_midlow),aprec(ind_emer_thr_midlow)...
    +0.25*MITSIM_a_Free_bra_midlow(ind_emer_thr_midlow,ind_emer_thr_midlow)...
    *oN(ind_emer_thr_midlow));
u(ind_emer_thr_mid) = min(MITSIM_a_Free_bra_mid(ind_emer_thr_mid,...
    ind_emer_thr_mid)*oN(ind_emer_thr_mid),aprec(ind_emer_thr_mid)...
    +0.25*MITSIM_a_Free_bra_mid(ind_emer_thr_mid,ind_emer_thr_mid)...
    *oN(ind_emer_thr_mid));
u(ind_emer_thr_midhigh) = min(MITSIM_a_Free_bra_midhigh(ind_emer_thr_midhigh,...
    ind_emer_thr_midhigh)*oN(ind_emer_thr_midhigh),aprec(ind_emer_thr_midhigh)...
    +0.25*MITSIM_a_Free_bra_midhigh(ind_emer_thr_midhigh,ind_emer_thr_midhigh)...
    *oN(ind_emer_thr_midhigh));
u(ind_emer_thr_high) = min(MITSIM_a_Free_bra_high(ind_emer_thr_high,...
    ind_emer_thr_high)*oN(ind_emer_thr_high),aprec(ind_emer_thr_high)...
    +0.25*MITSIM_a_Free_bra_high(ind_emer_thr_high,ind_emer_thr_high)...
    *oN(ind_emer_thr_high));
u(ind_emer_bra_low) = min(MITSIM_a_Free_bra_low(ind_emer_bra_low,...
    ind_emer_bra_low)*oN(ind_emer_bra_low),aprec(ind_emer_bra_low)...
    -0.5*(v(ind_emer_bra_low)-vprec(ind_emer_bra_low))...
    .^2./h(ind_emer_bra_low));
u(ind_emer_bra_midlow) = min(MITSIM_a_Free_bra_midlow(ind_emer_bra_midlow,...
    ind_emer_bra_midlow)*oN(ind_emer_bra_midlow),aprec(ind_emer_bra_midlow)...
    -0.5*(v(ind_emer_bra_midlow)-vprec(ind_emer_bra_midlow))...
    .^2./h(ind_emer_bra_midlow));
u(ind_emer_bra_mid) = min(MITSIM_a_Free_bra_mid(ind_emer_bra_mid,...
    ind_emer_bra_mid)*oN(ind_emer_bra_mid),aprec(ind_emer_bra_mid)...
    -0.5*(v(ind_emer_bra_mid)-vprec(ind_emer_bra_mid))...
    .^2./h(ind_emer_bra_mid));
u(ind_emer_bra_midhigh) = min(MITSIM_a_Free_bra_midhigh(ind_emer_bra_midhigh,...
    ind_emer_bra_midhigh)*oN(ind_emer_bra_midhigh),aprec(ind_emer_bra_midhigh)...
    -0.5*(v(ind_emer_bra_midhigh)-vprec(ind_emer_bra_midhigh))...
    .^2./h(ind_emer_bra_midhigh));
u(ind_emer_bra_high) = min(MITSIM_a_Free_bra_high(ind_emer_bra_high,...
    ind_emer_bra_high)*oN(ind_emer_bra_high),aprec(ind_emer_bra_high)...
    -0.5*(v(ind_emer_bra_high)-vprec(ind_emer_bra_high))...
    .^2./h(ind_emer_bra_high));
end

== matlab function A_Justo_SCHFV_slx_Track/IDM/MATLAB Function1 ==
  data: h input; v input; vprec input; IDM_T input; IDM_H0 input; IDM_V0 input; IDM_Amax input; IDM_Delta input; u output; IDM_iSqab input; oN input
function u = fcn(h,v,vprec,IDM_T,IDM_H0,IDM_V0,IDM_Amax,IDM_Delta,IDM_iSqab,oN)

% IDM
hr = IDM_H0+max(oN*0,IDM_T*v+v.*(v-vprec).*IDM_iSqab);
v = v.*(v>0); % Condition for avoiding numerical errors
% Control
u = IDM_Amax*(oN-(v./IDM_V0).^IDM_Delta-(hr./h).^2);

== matlab function A_Justo_SCHFV_slx_Track/Reference speeds/Distance control saturation ==
  data: v_r_0 input; T_s_0 input; h input; vprec input; IDM_H0 input; IDM_T input; v_r_1 output; acc1 input; acc2 input; v_r_2 output; T_s_1 output; T_s_2 output
function [v_r_1, v_r_2, T_s_1, T_s_2] = fcn(v_r_0, T_s_0, h, vprec, IDM_H0, IDM_T, acc1, acc2)

v_r_1 = v_r_0;
v_r_2 = v_r_0;
T_s_1 = T_s_0;
T_s_2 = T_s_0;

% if v_r_0 >= vprec(acc1)
%     v_r_1 = min(v_r_0, max(0, (h(acc1)-IDM_H0(acc1))/IDM_T(acc1,acc1)));
% end
% if v_r_0 >= vprec(acc2)
%     v_r_2 = min(v_r_0, max(0, (h(acc2)-IDM_H0(acc2))/IDM_T(acc2,acc2)));
% end

== matlab function A_Justo_SCHFV_slx_Track/Best stable R0 and R1 poles/Pole allocation #2 ==
  data: v_r input; P output; T_s input
function P = fcn(v_r, T_s) % He mirado en el gráfico una T_s que funcione bien, pero habría que calcularlo a partir de v_r
% Design of the control
M_p = 1e-10; %overshoot
sigma = 4/T_s; %real part of dominant pair
omega = -pi*sigma/log(M_p); %imaginary part of dominant pair
pDom = -sigma + 1i*omega;
pNeg1 = -21*sigma; pNeg2 = -22*sigma; pNeg3 = -23*sigma; pNeg4 = -24*sigma;
P = [pDom; conj(pDom); pNeg1; pNeg2; pNeg3; pNeg4];
%P = [-sigma; pNeg1; pNeg2; pNeg3; pNeg4; -25*sigma];
end

== matlab function A_Justo_SCHFV_slx_Track/Controller/Autonomous vehicle #1/Barrier ==
  data: h input; xb output; IDM_H0 input; acc1 input
function xb = fcn(h,IDM_H0,acc1)

h_min = 0.0;

%if h(acc1) < 3*IDM_H0(acc1)
    xb = 0.1/abs((h(acc1)-h_min))^1;
    %xb = -log(abs(h(acc1)-h_min));
    %xb = 1000/abs(h(acc1)-h_min)^0.1;
%else
%    xb = 0;
end

== matlab function A_Justo_SCHFV_slx_Track/Controller/Autonomous vehicle #2/Barrier ==
  data: h input; xb output; acc2 input
function xb = fcn(h,acc2)

h_min = 0.0;

if acc2 ~= 0
    xb = 0.1/abs((h(acc2)-h_min))^1;
else
    xb = 0;
end
end

== matlab function A_Justo_SCHFV_slx_Track/Controller/Autonomous vehicle #1/Gain scheduling ==
  data: kz output; v_r_0 input; K output; P input; IDM_Amax input; IDM_Bmax input; IDM_Delta input; Tau input; IDM_T input; IDM_H0 input; IDM_V0 input; acc1 input; n1 input
function [kz,K] = fcn(v_r_0,P,IDM_Amax,IDM_Bmax,IDM_Delta,Tau,IDM_T,IDM_H0,IDM_V0,acc1,n1)

% ACKERMANN'S FORMULA // STATE FEEDBACK WITH INTEGRAL ACTION

IDM_Amax = IDM_Amax(acc1+n1,acc1+n1);
IDM_Bmax = IDM_Bmax(acc1+n1,acc1+n1);
IDM_Delta = IDM_Delta(acc1+n1);
Tau_H = Tau(acc1+n1,acc1+n1);
Tau_A = Tau(acc1,acc1);
eta = IDM_T(acc1+n1,acc1+n1);
IDM_T = IDM_T(acc1+n1,acc1+n1);
IDM_H0 = IDM_H0(acc1+n1);
IDM_V0 = IDM_V0(acc1+n1);

A31 = 2*IDM_Amax/Tau_H/(IDM_H0+v_r_0*IDM_T)*(1-(v_r_0/IDM_V0)^IDM_Delta)^(3/2);
A32 = -IDM_Amax/Tau_H*(IDM_Delta*v_r_0^(IDM_Delta-1)/IDM_V0^IDM_Delta+(v_r_0+2*IDM_T*sqrt(IDM_Amax*IDM_Bmax))/((IDM_H0+v_r_0*IDM_T)*sqrt(IDM_Amax*IDM_Bmax))*(1-(v_r_0/IDM_V0)^IDM_Delta));
A34 = IDM_Amax/Tau_H*v_r_0/((IDM_H0+v_r_0*IDM_T)*sqrt(IDM_Amax*IDM_Bmax))*(1-(v_r_0/IDM_V0)^IDM_Delta);

% Linearized system
A = [ 0    -1     -eta      1       0    0 ;...
      0     0       1       0       0    0 ;...
     A31   A32  -1/Tau_H   A34      0    0 ;...
      0     0       0       0       1    0 ;...
      0     0       0       0   -1/Tau_A 0 ;...
      0     1       0       0       0    0 ];
B = [0; 0; 0; 0; 1/Tau_A; 0];

% Controllability matrix
W_C = [B A*B A^2*B A^3*B A^4*B A^5*B];

% Desired polynomial
P_d = (A-P(1)*eye(6))*(A-P(2)*eye(6))*(A-P(3)*eye(6))*(A-P(4)*eye(6))...
    *(A-P(5)*eye(6))*(A-P(6)*eye(6));

% Ackermann's formula
Kack = [0 0 0 0 0 1]*(W_C\P_d);
Kack = real(Kack);

% Gains
kz = Kack(6); K = [Kack(1) Kack(2) Kack(3) Kack(4) Kack(5)];
end
